simulink model "TV_2017"  (R2016a)
settings: Solver=FixedStepAuto  StartTime=0.0  StopTime=inf  FixedStep=0.001  RelTol=1e-3
PreLoadFcn:
  | TV_2017_parameters
values from neighbouring files (symbols this model uses):
  battery_voltage = single(530)    [HIL_parameters.m]    (also in HIL_parameters_2018.m; TV_2017_parameters.m; TV_2017_parameters_VD.m)
  car_params = Simulink_Car_params    [HIL_parameters.m]    (also in HIL_parameters_2018.m; TV_2017_parameters.m; TV_2017_parameters_VD.m)
  i_Diff = 16    [HIL_parameters.m]    (also in HIL_parameters_2018.m; TV_2017_parameters.m)
  Kp = 1    [HIL_parameters.m]    (also in HIL_parameters_2018.m; TV_2017_parameters.m; TV_2017_parameters_VD.m)
  motor_data = struct    [HIL_parameters.m]    (also in HIL_parameters_2018.m; TV_2017_parameters.m)
  powerLimitControl = Simulink_el    [HIL_parameters.m]    (also in HIL_parameters_2018.m; TV_2017_parameters.m; TV_2017_parameters_VD.m)
  settings = Simulink_Settings    [HIL_parameters.m]    (also in HIL_parameters_2018.m; TV_2017_parameters.m; TV_2017_parameters_VD.m)
  SpdC_BCC = 0    [HIL_parameters.m]    (also in HIL_parameters_2018.m; TV_2017_parameters.m; TV_2017_parameters_VD.m)
  Speed_Neg_sat = -21    [HIL_parameters.m]    (also in HIL_parameters_2018.m; TV_2017_parameters.m; TV_2017_parameters_VD.m)
  Speed_Pos_sat = 21    [HIL_parameters.m]    (also in HIL_parameters_2018.m; TV_2017_parameters.m; TV_2017_parameters_VD.m)
  SteeringAngleFL = [-23.80 -22.65 -21.50 -20.34 -19.18 -18.03 -16.86 -15.70 -14.53 -13.35 -12.18 -10.99 -9.80 -8.61 -7.40 -6.19 -4.97 -3.75 -2.51 -1.26 0 1.27 2.56 3.85 5.17 6.50 7.84 9.21 10.59 12.00 13.42 14.88 16.36 17.87 19.41 20.99 22.61 24.26 25.97 27.73 29.54]    [CarSetupAnalysis2018.m]    (also in HIL_parameters_2018.m; TV_2017_parameters.m; TV_2017_parameters_VD.m = [-24.129 -22.950 -21.772 -20.593 -19.413 -18.232 -17.050 -15)
  SteeringAngleFR = [-29.54 -27.73 -25.97 -24.26 -22.61 -20.99 -19.41 -17.87 -16.36 -14.88 -13.42 -12.00 -10.59 -9.21 -7.84 -6.50 -5.17 -3.85 -2.56 -1.27 0 1.26 2.51 3.75 4.97 6.19 7.40 8.61 9.80 10.99 12.18 13.35 14.53 15.70 16.86 18.03 19.18 20.34 21.50 22.65 23.80]    [CarSetupAnalysis2018.m]    (also in HIL_parameters_2018.m; TV_2017_parameters.m; TV_2017_parameters_VD.m = [-29.3050 -27.5340 -25.8140 -24.1410 -22.5110 -20.9180 -19.3)
  SteeringWhAngle = [-105 -99.75 -94.5 -89.25 -84 -78.75 -73.5 -68.25 -63 -57.75 -52.5 -47.25 -42 -36.75 -31.5 -26.25 -21.0 -15.75 -10.5 -5.25 0.0 5.25 10.50 15.75 21.00 26.25 31.50 36.75 42.00 47.25 52.50 57.75  63.00 68.25 73.50 78.75 84.00 89.25 94.50 99.75 105.00]    [TV_2017_parameters_VD.m]
  Tn_n = 0    [HIL_parameters.m]    (also in HIL_parameters_2018.m; TV_2017_parameters.m; TV_2017_parameters_VD.m)
  tractionControl = Simulink_tc    [HIL_parameters.m]    (also in HIL_parameters_2018.m; IterativeTractionControlTuning.m; TV_2017_parameters.m; TV_2017_parameters_VD.m)
  yawMomentGenerator = struct    [HIL_parameters.m]    (also in HIL_parameters_2018.m = Simulink_yawRate2; TV_2017_parameters.m = Simulink_yawRate2)
  yawRateControl = Simulink_yawRate    [HIL_parameters.m]    (also in HIL_parameters_2018.m; TV_2017_parameters.m; TV_2017_parameters_VD.m)
undefined symbols (not defined in the file or in its folder): DiscIntNeverNeededParam, magnitude, speedEstimation, TC_Decr_Gas, TC_Derivative, TC_Incr_Gas, TC_On, TC_Relay_Off, TC_Relay_On
libraries: CarMaker4SL x350, simulink_extras x63, simulink x37, dspfdesign x2
(part 8 of 14)

== system TV_2017/CarMaker/IPG Vehicle3/PowerTrain/Electric Powertrain/E-Gas // E-Motor/Electronic Gas Pedal RR/Subsystem1 ==
  VC.Gas : Inport
  E_Gas. : Inport  Port=2
  Car.LongSlip : Inport  Port=3
  Add : Sum
  Compare To Constant : simulink/Logic and Bit Operations/Compare To Constant  relop=>  const=TC_Derivative  OutDataTypeStr=uint8  ZeroCross=off
  Derivative : Derivative
  Fcn : Fcn  Expr=u >0.05
  Fcn1 : Fcn  Expr=u+TC_Incr_Gas
  Fcn2 : Fcn  Expr=u-TC_Decr_Gas
  Multiport Switch : MultiPortSwitch  DataPortOrder=Zero-based contiguous  zeroidx=on
  Relational Operator : RelationalOperator  Operator=<=  InputSameDT=on
  Relay : Relay  OnSwitchValue=TC_Relay_On  OffSwitchValue=TC_Relay_Off
  S-R Flip-Flop : simulink_extras/Flip Flops/S-R Flip-Flop  initial_condition=0
  Saturation : Saturate  UpperLimit=1  LowerLimit=0
  Saturation1 : Saturate  UpperLimit=1  LowerLimit=0
  Switch : Switch  Criteria=u2 > Threshold
  Terminator : Terminator
  E_Gas : Outport
  wires:
  Car.LongSlip/1 -> Relay/1, Derivative/1, Fcn/1
  Relay/1 -> Add/1
  Derivative/1 -> Compare To Constant/1
  Compare To Constant/1 -> Add/2
  Add/1 -> Multiport Switch/1
  Multiport Switch/1 -> E_Gas/1
  VC.Gas/1 -> Relational Operator/1, [A]
  E_Gas./1 -> Relational Operator/2, Fcn1/1, Fcn2/1, Multiport Switch/3
  S-R Flip-Flop/2 -> Terminator/1
  S-R Flip-Flop/1 -> Switch/2
  Switch/1 -> Multiport Switch/2
  Fcn/1 -> S-R Flip-Flop/1
  Relational Operator/1 -> S-R Flip-Flop/2
  Fcn1/1 -> Saturation1/1
  Saturation1/1 -> Switch/1
  Fcn2/1 -> Saturation/1
  Saturation/1 -> Multiport Switch/4
  [A] -> Switch/3

== matlab function TV_2017/CarMaker/Control_System /Yaw_rate_Mz_generator/Yaw Rate Controller /yawRateReference ==
  data: r_der_error output; r_error output; vx output; states input Bus: States; prev_r_error input; r_ref output; yawRateControl parameter; car_params parameter; r_lim output; settings parameter
function [r_der_error,r_error, vx, r_ref,r_lim]...
          = yawrate_reference(states,prev_r_error, yawRateControl, car_params,settings)

%#codegen
updatefactor = single(1);
r_lim = single(0);
delta = states.wheel_angle;
delta_der = states.wheel_speed;
% If Ku is negative there will be a problem if the denominator approaches
% zero at high speeds
r_ref = (states.V_x/(yawRateControl.r_ref_tuning_param + yawRateControl.Ku*states.V_x^2))*tan(delta); %  tan

%r_ref = (states.V_x/(yawRateControl.r_ref_tuning_param*(1 + yawRateControl.Ku*states.V_x^2)))* delta;

%Fzi = [states.Fz_FL states.Fz_FR states.Fz_RL states.Fz_RR];
if yawRateControl.enable_r_ref_limit == 1
    r_lim = settings.mu*yawRateControl.mu_scaling_r_ref_limit*9.81/states.V_x;
    if abs(r_ref) > abs(r_lim)
        r_ref = r_lim*sign(r_ref);
    end
end

r = states.r;
r_error = prev_r_error*(1-updatefactor) + updatefactor*(r_ref-r);
r_ref_der = (states.ax*delta + states.V_x*delta_der)/yawRateControl.r_ref_tuning_param;
r_der_error = r_ref_der*yawRateControl.ref_weight - states.r_der*yawRateControl.meas_weight;

vx = states.V_x;
end

== matlab function TV_2017/CarMaker/Control_System /Slip Rate Control /Traction Controllers/MATLAB Function1 ==
  data: states input Bus: States; SR_FL output; SR_FR output; SR_RL output; SR_RR output; T_req input; tractionControl parameter; Kp output; Ki output; settings parameter; T_tv input Bus: Ti_lim
function [SR_FL, SR_FR, SR_RL, SR_RR, Kp, Ki] = slipRatioAndGains(states, T_req, tractionControl, settings, T_tv)
%#codegen


SR_FL = states.SR_FL;
SR_FR = states.SR_FR;
SR_RL = states.SR_RL;
SR_RR = states.SR_RR;



if (states.V_x >= 0) 
    vx_kmh = states.V_x*3.6;
else
    vx_kmh = single(0);
end

    

a_kp = single((tractionControl.Kp_end - tractionControl.Kp_start) / tractionControl.lookup_speed_end_kmh);
a_ki = single((tractionControl.Ki_end - tractionControl.Ki_start) / tractionControl.lookup_speed_end_kmh);



if ( ( (T_req + 0.0001) > 0) && (vx_kmh < tractionControl.full_gain_limit_kmh) )   
    Kp = min( (a_kp*max(0,vx_kmh) + tractionControl.Kp_start), tractionControl.Kp_end)  * abs(T_req)/(settings.max_motor_torque*4);
    Ki = min( (a_ki*max(0,vx_kmh) + tractionControl.Ki_start), tractionControl.Ki_end)  * abs(T_req)/(settings.max_motor_torque*4);
else
    Kp = min( (a_kp*max(0,vx_kmh) + tractionControl.Kp_start), tractionControl.Kp_end);
    Ki = min( (a_ki*max(0,vx_kmh) + tractionControl.Ki_start), tractionControl.Ki_end);
end

end






% This one solves starting from 0 kmh with the driver controlling the
% throttle. This statement reduces the gains according to the requested
% torque, to avoid oscillating torque output


% if ( ( (T_req + 0.0001) > 0) && (vx_kmh < tractionControl.full_gain_limit_kmh) )   
%     Kp_driving = min( (a_kp*max(0,vx_kmh) + tractionControl.Kp_start), tractionControl.Kp_end)  * abs(T_req)/(settings.max_motor_torque*4);
%     Ki_driving = min( (a_ki*max(0,vx_kmh) + tractionControl.Ki_start), tractionControl.Ki_end)  * abs(T_req)/(settings.max_motor_torque*4);
%     Kp_FL = Kp_driving;
%     Kp_FR = Kp_driving;
%     Kp_RL = Kp_driving;
%     Kp_RR = Kp_driving;
%     
%     Ki_FL = Ki_driving;
%     Ki_FR = Ki_driving;
%     Ki_RL = Ki_driving;
%     Ki_RR = Ki_driving;
%     %Kp = min( (a_kp*max(0,vx_kmh) + tractionControl.Kp_start), tractionControl.Kp_end)  * abs(T_req)/(settings.max_motor_torque*4);
%     %Ki = min( (a_ki*max(0,vx_kmh) + tractionControl.Ki_start), tractionControl.Ki_end)  * abs(T_req)/(settings.max_motor_torque*4);
% 
% % T_req positive and speed over full gain limit
% elseif ( ( (T_req + 0.0001) > 0) && (vx_kmh > tractionControl.full_gain_limit_kmh))
%     Kp_driving = min( (a_kp*max(0,vx_kmh) + tractionControl.Kp_start), tractionControl.Kp_end);
%     Ki_driving = min( (a_ki*max(0,vx_kmh) + tractionControl.Ki_start), tractionControl.Ki_end);
%     Kp_FL = Kp_driving;
%     Kp_FR = Kp_driving;
%     Kp_RL = Kp_driving;
%     Kp_RR = Kp_driving;
%     
%     Ki_FL = Ki_driving;
%     Ki_FR = Ki_driving;
%     Ki_RL = Ki_driving;
%     Ki_RR = Ki_driving;    
% else   
%     Kp_FL = min( (a_kp*max(0,vx_kmh) + tractionControl.Kp_start), tractionControl.Kp_end);
%     Kp_FR = min( (a_kp*max(0,vx_kmh) + tractionControl.Kp_start), tractionControl.Kp_end);
%     Kp_RL = min( (a_kp*max(0,vx_kmh) + tractionControl.Kp_start), tractionControl.Kp_end);
%     Kp_RR = min( (a_kp*max(0,vx_kmh) + tractionControl.Kp_start), tractionControl.Kp_end);
%     
%     Ki_FL = min( (a_ki*max(0,vx_kmh) + tractionControl.Ki_start), tractionControl.Ki_end);
%     Ki_FR = min( (a_ki*max(0,vx_kmh) + tractionControl.Ki_start), tractionControl.Ki_end);
%     Ki_RL = min( (a_ki*max(0,vx_kmh) + tractionControl.Ki_start), tractionControl.Ki_end);
%     Ki_RR = min( (a_ki*max(0,vx_kmh) + tractionControl.Ki_start), tractionControl.Ki_end);
%     
%     %Kp = tractionControl.Kp_braking;
%     %Ki = tractionControl.Ki_braking;
% end
% 
% if ( (T_tv.FL < 0) || (T_tv.FR < 0) || (T_tv.RL < 0) || (T_tv.RR < 0) )
%     Kp = tractionControl.Kp_braking;
%     Ki = tractionControl.Ki_braking;
% end

== matlab function TV_2017/CarMaker/Control_System /MATLAB Function3 ==
  data: Ti input Bus: Ti_lim; states input; Ti_pos output Bus: Ti_pos; Ti_neg output Bus: Ti_neg; wi_setpoints output Bus: wi_set; settings parameter; car_params parameter; overTorque output
function [Ti_pos, Ti_neg, wi_setpoints, overTorque] = setPointCalculation(Ti,states,settings,car_params)
%#codegen

%Conversion factor to calculate RPM limits based on speed limits
%v_to_motor_RPM = single(60*car_params.GR/(2*pi*car_params.r_eff));
overTorque = int8(0);
r = car_params.r_eff;
GR = car_params.GR;
scale_factor = 5;
not_in_use = settings.RPM_scaling;
max_rpm = settings.max_RPM;
KERS_RPM_setpoint = settings.KERS_motor_RPM_setpoint;
%scaled_RPM_lim_pos = states.V_x* (60/2*pi*r)*scale_factor;
v_x = states.V_x;
if v_x>5;
    scaled_RPM_lim_pos =  min([max_rpm ,GR*v_x* (60/2*pi*r)*scale_factor]);
else
   scaled_RPM_lim_pos = single( min([max_rpm ,GR*5* (60/2*pi*r)*scale_factor]));
end


if max([Ti.FL Ti.FR Ti.RL Ti.RR]) > (21+0.0001)
    %this is bad
    overTorque = int8(1);
end



 %***************** FL *********** 

if  (Ti.FL <= 0)  
    Ti_pos.FL = int16(0);
    Ti_neg.FL = int16(max(-settings.max_motor_brake_torque/car_params.Mn, Ti.FL/car_params.Mn));
    wi_setpoints.FL = int16(KERS_RPM_setpoint);

elseif Ti.FL > 0
    Ti_pos.FL = int16(min(21/car_params.Mn , Ti.FL/car_params.Mn));
    Ti_neg.FL = int16(0);
    wi_setpoints.FL = int16(max_rpm);  
else
    Ti_pos.FL = int16(0);
    Ti_neg.FL = int16(0);
    wi_setpoints.FL = int16(1); 
end

%***************** FR ************

if  (Ti.FR <= 0)
    Ti_pos.FR = int16(0);
    Ti_neg.FR = int16(max(-settings.max_motor_brake_torque/car_params.Mn, Ti.FR/car_params.Mn));
    wi_setpoints.FR = int16(KERS_RPM_setpoint);

elseif Ti.FR > 0        
    Ti_pos.FR = int16( min(21/car_params.Mn , Ti.FR/car_params.Mn));
    Ti_neg.FR = int16(0);
    wi_setpoints.FR = int16(max_rpm);  
else
    Ti_pos.FR = int16(0);
    Ti_neg.FR = int16(0);
    wi_setpoints.FR = int16(1); 
end
%***************** RL ************
if  (Ti.RL <= 0)
    Ti_pos.RL = int16(0);
    Ti_neg.RL = int16(max(-settings.max_motor_brake_torque/car_params.Mn, Ti.RL/car_params.Mn));
    wi_setpoints.RL = int16(KERS_RPM_setpoint);

elseif Ti.RL > 0
    Ti_pos.RL = int16(min(21/car_params.Mn , Ti.RL/car_params.Mn));
    Ti_neg.RL = int16(0);
    wi_setpoints.RL = int16(max_rpm);  
else
    Ti_pos.RL = int16(0);
    Ti_neg.RL = int16(0);
    wi_setpoints.RL = int16(1); 
end

%***************** RR ************
if (Ti.RR <= 0)
    Ti_pos.RR = int16(0);
    Ti_neg.RR = int16(max(-settings.max_motor_brake_torque/car_params.Mn, Ti.RR/car_params.Mn));
    wi_setpoints.RR = int16(KERS_RPM_setpoint);

elseif Ti.RR > 0
    Ti_pos.RR = int16(min(21/car_params.Mn , Ti.RR/car_params.Mn));
    Ti_neg.RR = int16(0);
    wi_setpoints.RR = int16(max_rpm);  
else
    Ti_pos.RR = int16(0);
    Ti_neg.RR = int16(0);
    wi_setpoints.RR = int16(1); 
end
end



% _________________________________________________________________________________________  
% 
% %***************** FL ************
% if dynamic_rpm ==1
%     if  (Ti.FL <= 0)  
%         Ti_pos.FL = int16(0);
%         Ti_neg.FL = int16(max(-settings.max_motor_brake_torque/car_params.Mn, Ti.FL/car_params.Mn));
%         wi_setpoints.FL = int16(KERS_RPM_setpoint);
% 
%     elseif Ti.FL > 0 
%         Ti_pos.FL = int16( Ti.FL/car_params.Mn);
%         Ti_neg.FL = int16(0);
%         wi_setpoints.FL = int16(scaled_RPM_lim_pos);  
%     else
%         Ti_pos.FL = int16(0);
%         Ti_neg.FL = int16(0);
%         wi_setpoints.FL = int16(2); 
%     end
% 
%     %***************** FR ************
% 
%     if  (Ti.FR <= 0)
%         Ti_pos.FR = int16(0);
%         Ti_neg.FR = int16(max(-settings.max_motor_brake_torque/car_params.Mn, Ti.FR/car_params.Mn));
%         wi_setpoints.FR = int16(KERS_RPM_setpoint);
% 
%     elseif Ti.FR > 0
%         Ti_pos.FR = int16( Ti.FR/car_params.Mn);
%         Ti_neg.FR = int16(0);
%         wi_setpoints.FR = int16(scaled_RPM_lim_pos);  
%     else
%         Ti_pos.FR = int16(0);
%         Ti_neg.FR = int16(0);
%         wi_setpoints.FR = int16(2); 
%     end
%     %***************** RL ************
%     if  (Ti.RL <= 0)
%         Ti_pos.RL = int16(0);
%         Ti_neg.RL = int16(max(-settings.max_motor_brake_torque/car_params.Mn, Ti.RL/car_params.Mn));
%         wi_setpoints.RL = int16(KERS_RPM_setpoint);
% 
%     elseif Ti.RL > 0
%         Ti_pos.RL = int16( Ti.RL/car_params.Mn);
%         Ti_neg.RL = int16(0);
%         wi_setpoints.RL = int16(scaled_RPM_lim_pos);  
%     else
%         Ti_pos.RL = int16(0);
%         Ti_neg.RL = int16(0);
%         wi_setpoints.RL = int16(2); 
%     end
% 
%     %***************** RR ************
%     if (Ti.RR <= 0)
%         Ti_pos.RR = int16(0);
%         Ti_neg.RR = int16(max(-settings.max_motor_brake_torque/car_params.Mn, Ti.RR/car_params.Mn));
%         wi_setpoints.RR = int16(KERS_RPM_setpoint);
% 
%     elseif Ti.RR > 0
%         Ti_pos.RR = int16( Ti.RR/car_params.Mn);
%         Ti_neg.RR = int16(0);
%         wi_setpoints.RR = int16(scaled_RPM_lim_pos);  
%     else
%         Ti_pos.RR = int16(0);
%         Ti_neg.RR = int16(0);
%         wi_setpoints.RR = int16(2); 
%     end
%     
%     
% else
%     
%     
    
  % _________________________________________________________________________________________  
% % The RPM at which KERS is turned off
% RPM_limit_low = settings.KERS_speed_limit_hyst_low*v_to_motor_RPM;
% 
% % The RPM at which KERS is allowed again
% RPM_limit_high = settings.KERS_speed_limit_hyst_high*v_to_motor_RPM;
% 
% 
%    persistent firstIteration;
%    persistent KERS_ALLOWED_FL;
%    persistent KERS_ALLOWED_FR;
%    persistent KERS_ALLOWED_RL;
%    persistent KERS_ALLOWED_RR;
%    
%    
%    % Hysteresis on regenerative input based on RPM to avoid oscillation around 
%    % allowed KERS RPM 
%    if isempty(firstIteration)
%       firstIteration = 2; % Avoid overflow in the register and count 1 again
%       KERS_ALLOWED_FL = uint32(0);
%       KERS_ALLOWED_FR = uint32(0);
%       KERS_ALLOWED_RL = uint32(0);
%       KERS_ALLOWED_RR = uint32(0);
%    else
%        
%        %Hysteris around the minimum RPM Set point
%        if     ( (KERS_ALLOWED_FL == 0) && (states.RPM_FL > RPM_limit_high) )
%            KERS_ALLOWED_FL = uint32(1);
%        elseif ( (KERS_ALLOWED_FL == 1) && (states.RPM_FL < RPM_limit_low) )
%            KERS_ALLOWED_FL = uint32(0);
%        end
%        if     ( (KERS_ALLOWED_FR == 0) && (states.RPM_FR > RPM_limit_high) )
%            KERS_ALLOWED_FR = uint32(1);
%        elseif ( (KERS_ALLOWED_FR == 1) && (states.RPM_FR < RPM_limit_low) )
%            KERS_ALLOWED_FR = uint32(0);
%        end
%        if     ( (KERS_ALLOWED_RL == 0) && (states.RPM_RL > RPM_limit_high) )
%            KERS_ALLOWED_RL = uint32(1);
%        elseif ( (KERS_ALLOWED_RL == 1) && (states.RPM_RL < RPM_limit_low) )
%            KERS_ALLOWED_RL = uint32(0);
%        end
%        if     ( (KERS_ALLOWED_RR == 0) && (states.RPM_RR > RPM_limit_high) )
%            KERS_ALLOWED_RR = uint32(1);
%        elseif ( (KERS_ALLOWED_RR == 1) && (states.RPM_RR < RPM_limit_low) )
%            KERS_ALLOWED_RR = uint32(0);
%        end
%        
%        % Hysteresis around maximum RPM ? 
%        
%    end   
%       
% %***************** FL ************
% 
% if ( (Ti.FL <= 0) && (KERS_ALLOWED_FL == 1) ) 
%     Ti_pos.FL = int16(0);
%     Ti_neg.FL = int16( Ti.FL/car_params.Mn);
%     wi_setpoints.FL = int16(KERS_RPM_setpoint);
% elseif ( (Ti.FL <= 0) && (KERS_ALLOWED_FL == 0) )
%     Ti_pos.FL = int16(0);
%     Ti_neg.FL = int16(0);
%     wi_setpoints.FL = int16(0);
% elseif Ti.FL > 0
%     Ti_pos.FL = int16( Ti.FL/car_params.Mn);
%     Ti_neg.FL = int16(0);
%     wi_setpoints.FL = int16(max_rpm);  
% else
%     Ti_pos.FL = int16(0);
%     Ti_neg.FL = int16(0);
%     wi_setpoints.FL = int16(0); 
% end
% 
% %***************** FR ************
% 
% if ( (Ti.FR <= 0) && (KERS_ALLOWED_FR == 1) ) 
%     Ti_pos.FR = int16(0);
%     Ti_neg.FR = int16( Ti.FR/car_params.Mn);
%     wi_setpoints.FR = int16(KERS_RPM_setpoint);
% elseif ( (Ti.FR <= 0) && (KERS_ALLOWED_FR == 0) )
%     Ti_pos.FR = int16(0);
%     Ti_neg.FR = int16(0);
%     wi_setpoints.FR = int16(0);
% elseif Ti.FR > 0
%     Ti_pos.FR = int16( Ti.FR/car_params.Mn);
%     Ti_neg.FR = int16(0);
%     wi_setpoints.FR = int16(max_rpm);  
% else
%     Ti_pos.FR = int16(0);
%     Ti_neg.FR = int16(0);
%     wi_setpoints.FR = int16(0); 
% end
% %***************** RL ************
% if ( (Ti.RL <= 0) && (KERS_ALLOWED_RL == 1) ) 
%     Ti_pos.RL = int16(0);
%     Ti_neg.RL = int16( Ti.RL/car_params.Mn);
%     wi_setpoints.RL = int16(KERS_RPM_setpoint);
% elseif ( (Ti.RL <= 0) && (KERS_ALLOWED_RL == 0) )
%     Ti_pos.RL = int16(0);
%     Ti_neg.RL = int16(0);
%     wi_setpoints.RL = int16(0);
% elseif Ti.RL > 0
%     Ti_pos.RL = int16( Ti.RL/car_params.Mn);
%     Ti_neg.RL = int16(0);
%     wi_setpoints.RL = int16(max_rpm);  
% else
%     Ti_pos.RL = int16(0);
%     Ti_neg.RL = int16(0);
%     wi_setpoints.RL = int16(0); 
% end
% 
% %***************** RR ************
% if ( (Ti.RR <= 0) && (KERS_ALLOWED_RR == 1) ) 
%     Ti_pos.RR = int16(0);
%     Ti_neg.RR = int16( Ti.RR/car_params.Mn);
%     wi_setpoints.RR = int16(KERS_RPM_setpoint);
% elseif ( (Ti.RR <= 0) && (KERS_ALLOWED_RR == 0) )
%     Ti_pos.RR = int16(0);
%     Ti_neg.RR = int16(0);
%     wi_setpoints.RR = int16(0);
% elseif Ti.RR > 0
%     Ti_pos.RR = int16( Ti.RR/car_params.Mn);
%     Ti_neg.RR = int16(0);
%     wi_setpoints.RR = int16(max_rpm);  
% else
%     Ti_pos.RR = int16(0);
%     Ti_neg.RR = int16(0);
%     wi_setpoints.RR = int16(0); 
% end
% 
% end

== matlab function TV_2017/CarMaker/Control_System /Yaw_rate_Mz_generator/Yaw Rate Controller /gainScheduling ==
  data: Kd output; vx_kmh input; Kp output; Ki output; yawRateControl parameter
function [Kd, Kp, Ki] = gainScheduling(vx_kmh,yawRateControl)
%#codegen
if (vx_kmh <= 0)
    vx_kmh = single(0);
end


% a_kp = single((yawRateControl.Kp_end - yawRateControl.Kp_start) / yawRateControl.lookup_speed_end_kmh);
% a_ki = single((yawRateControl.Ki_end - yawRateControl.Ki_start) / yawRateControl.lookup_speed_end_kmh);
% a_kd = single((yawRateControl.Kd_end - yawRateControl.Kd_start) / yawRateControl.lookup_speed_end_kmh);
% 
% if (vx_kmh <= 0)
%     vx_kmh = single(0);
% end
% 
% Kp = min( (a_kp*max(0.1,vx_kmh) + yawRateControl.Kp_start), yawRateControl.Kp_end);
% 
% Ki = min( (a_ki*max(0.1,vx_kmh) + yawRateControl.Ki_start), yawRateControl.Ki_end);
% 
% Kd = min( (a_kd*max(0.1,vx_kmh) + yawRateControl.Kd_start), yawRateControl.Kd_end);
% 
% end

Kp_values = [yawRateControl.Kp_start yawRateControl.Kp_start  yawRateControl.Kp_end yawRateControl.Kp_end];
Kp_speeds = [0 yawRateControl.lookup_speed_end_kmh (yawRateControl.lookup_speed_end_kmh+20)  115];

Ki_values = [yawRateControl.Ki_start yawRateControl.Ki_start  yawRateControl.Ki_end yawRateControl.Ki_end];
Ki_speeds = [0 yawRateControl.lookup_speed_end_kmh (yawRateControl.lookup_speed_end_kmh+20)  115];

Kd_values = [yawRateControl.Kd_start yawRateControl.Kd_start  yawRateControl.Kd_end yawRateControl.Kd_end];
Kd_speeds = [0 yawRateControl.lookup_speed_end_kmh (yawRateControl.lookup_speed_end_kmh+20)  115];


Kp = interp1(Kp_speeds,Kp_values,vx_kmh); 
Ki = interp1(Ki_speeds,Ki_values,vx_kmh);
Kd = interp1(Kd_speeds,Kd_values,vx_kmh);


if Kp>= 0
    Kp = Kp;
elseif Kp < 0 
    Kp = Kp;
else
    Kp = single(0);
end

if Ki>= 0
    Ki = Ki;
elseif Ki < 0 
    Ki = Ki;
else
    Ki = single(0);
end

if Kd>= 0
    Kd = Kd;
elseif Kd < 0 
    Kd = Kd;
else
    Kd = single(0);
end



breakpoint = 1;

== matlab function TV_2017/CarMaker/Control_System /Subsystem/OutputTelemetri ==
  data: states input; OutputTelemetri_control output Bus: OutputTelemetri_Control; T_req input; r_ref input; Mz_ref_to_telemetry input
function OutputTelemetri_control = OutputTelemetri(states, T_req, r_ref, Mz_ref_to_telemetry)
%#codegen

OutputTelemetri_control.T_req   = T_req;
OutputTelemetri_control.Mz_ref  = Mz_ref_to_telemetry;
OutputTelemetri_control.r_ref   = r_ref;
end

== matlab function TV_2017/CarMaker/Control_System /Subsystem/Torque allocation 2017/Inverter temperature limiter ==
  data: states input; maxMotorTorque output Bus: maxMotorTorque; settings parameter; car_params parameter
function maxMotorTorque = maxMotorTorque_InvTemp(states,settings, car_params)
%#codegen
inv_FL_temp =int16(20);
inv_FR_temp =20;
inv_RL_temp =20;
inv_RR_temp =20;


% The inverters limits output torque based on internal temperature
mmt                 =  single(settings.max_motor_torque);
upper_max_temp      =  single(car_params.AMK_inverter_upper_max_temp);
cutoff_temp         =  single(car_params.AMK_inverter_cutoff_temp);

torque = [mmt, mmt, single(0)]; %breakpoints for lookup function
temp = [single(0), upper_max_temp, cutoff_temp];

inv_FL_temp = single(states.AMK_inverter_temp_FL);
inv_FR_temp = single(states.AMK_inverter_temp_FR);
inv_RL_temp = single(states.AMK_inverter_temp_RL);
inv_RR_temp = single(states.AMK_inverter_temp_RR);

%  y = interp1(xdata,ydata,x)
maxMotorTorque.mmt_FL = interp1(  temp , torque,  inv_FL_temp  );
maxMotorTorque.mmt_FR = interp1(  temp , torque,  inv_FR_temp  );
maxMotorTorque.mmt_RL = interp1(  temp , torque,  inv_RL_temp  );
maxMotorTorque.mmt_RR = interp1(  temp , torque,  inv_RR_temp  );

== matlab function TV_2017/CarMaker/ECU input Sensors /estimated "Measured Power" based on Torque, RPM and datasheet IRL this is measured/MATLAB Function ==
  data: RPM_FL_IN input; RPM_FR_IN input; RPM_RL_IN input; RPM_RR_IN input; Pm_FL output; T input; T_FL output; RPM_FL output; Pm_FR output; T_FR output; RPM_FR output; Pm_RL output; T_RL output; RPM_RL output; Pm_RR output; T_RR output; RPM_RR output
function [Pm_FL, T_FL, RPM_FL,Pm_FR, T_FR, RPM_FR,Pm_RL, T_RL,...
          RPM_RL,Pm_RR, T_RR, RPM_RR] = powerMeasurement(RPM_FL_IN, RPM_FR_IN,RPM_RL_IN,RPM_RR_IN, T)
%#codegen

%Conversion from RPM to rad/s
c = single(2*pi/60);

T_FL = T.FL;
T_FR = T.FR;
T_RL = T.RL;
T_RR = T.RR;

RPM_FL = RPM_FL_IN;
RPM_FR = RPM_FR_IN;
RPM_RL = RPM_RL_IN;
RPM_RR = RPM_RR_IN;


Pm_FL = RPM_FL*c*T.FL;
Pm_FR = RPM_FR*c*T.FR;
Pm_RL = RPM_RL*c*T.RL;
Pm_RR = RPM_RR*c*T.RR;

== matlab function TV_2017/CarMaker/Control_System /Subsystem/Torque allocation 2016/MATLAB Function ==
  data: states input; maxMotorTorque output Bus: maxMotorTorque; settings parameter
function maxMotorTorque = findMaxMotorTorque(states,settings)
%#codegen

% DC Voltage                             / states
% Max allowable current draw in total    /settings
% Load distribution                      /states

Fzi = [max(1,states.Fz_FL) max(1,states.Fz_FR) max(1,states.Fz_RL) max(1,states.Fz_RR)]';

switch settings.TV_Method
    case 1 % No negative torque
        alfa_r =  (Fzi(3) + Fzi(4)) / (Fzi(1) + Fzi(2) + Fzi(3) + Fzi(4));
    case 2 % with negative torque
        alfa_r =  (Fzi(3) + Fzi(4)) / (Fzi(1) + Fzi(2) + Fzi(3) + Fzi(4));
    case 3 % static 25 %
        alfa_r = single(0.5);
    case 4 % with negative torque, no Fz
        alfa_r = single(0.5);
    otherwise
        alfa_r = single(0.5);
end

RPM_to_angular = single(2*pi/60);
omega_FL = states.RPM_FL*RPM_to_angular;
omega_FR = states.RPM_FR*RPM_to_angular;
omega_RL = states.RPM_RL*RPM_to_angular;
omega_RR = states.RPM_RR*RPM_to_angular;

mmt = settings.max_motor_torque;
available_power = states.DC_voltage*settings.max_battery_discharge;

max_torque_front = min(mmt, (available_power*(1-alfa_r))/ (2 * max( max(1,omega_FL), max(1,omega_FR))) );
max_torque_rear = min(mmt, (available_power*alfa_r)     / (2 * max( max(1,omega_RL), max(1,omega_RR))) );
                      
maxMotorTorque.mmt_FL = max_torque_front;
maxMotorTorque.mmt_FR = max_torque_front;
maxMotorTorque.mmt_RL = max_torque_rear;
maxMotorTorque.mmt_RR = max_torque_rear;
maxMotorTorque.kers_allowed = single(0);

== matlab function TV_2017/CarMaker/Estimations/EstimateVx/velocity_Estimation ==
  data: sensors input Bus: SensorInputs; V_est_x output; normalForces input Bus: normalForces; settings parameter; car_params parameter; speedEstimation parameter
function V_est_x  = velocityEstimation(sensors,normalForces,settings,car_params,speedEstimation)
%#codegen


persistent firstIteration;
persistent v;
persistent error;
persistent K;
persistent drift;

k_FL = single(0); % Gain 
k_FR = single(0); % Gain
k_RL = single(0); % Gain
k_RR = single(0); % Gain
% Gains for trusting, not trusting wheel speed measurements
Hg = speedEstimation.High_gain;
Lg = speedEstimation.Low_gain;
% Variances
all_Var = single(0); % Variance for all measurements
front_rear_Var = single(0);
front_Var = single(0);
rear_Var = single(0);
left_Var = single(0);
right_Var = single(0);
% LIMITS:
velocity_deviation_limit = speedEstimation.velocity_deviation_limit;
lim = speedEstimation.variance_limit;
RPM_derivative_limit = speedEstimation.RPM_derivative_limit;

% Measurement vector
C = [1;1;1;1]; % Create four copies of predicted vx


c = single(2*pi/(car_params.GR*60));

t = settings.control_system_sample_time;
%Weights taken from wikipedia
%sg_Weight = single( [ 1; -8; 0; 8; -1] );
sg_Weight = single( [ -1; 8; 0; -8; 1] );
%sg_Weight = single([0.3; 0.1; -0.1 ; -0.3]);
%sg_Weight = single([1; -1; 0 ; -0]);
% ------------------------------
% COPY VARIABLES EACH TIMESTEP
% ------------------------------
S = sensors.steering_wheel_angle; % Steering angle in rad( Mean of front wheels)
ax = sensors.ax; % Should be true linear acceleration compensated for roll angle
%Fz, used to determine what wheel speeds to trust.
Fz = [normalForces.FL, normalForces.FR, normalForces.RL ,normalForces.RR];
% Determine CoG Vx from motor RPM. Simple atm. Not considering vy.
Whl_v_FL = sensors.RPM_FL*c*car_params.r_eff*cos(S) + sensors.yawRate*car_params.t_f;
Whl_v_FR = sensors.RPM_FR*c*car_params.r_eff*cos(S) - sensors.yawRate*car_params.t_f;
Whl_v_RL = sensors.RPM_RL*c*car_params.r_eff + sensors.yawRate*car_params.t_r;
Whl_v_RR = sensors.RPM_RR*c*car_params.r_eff - sensors.yawRate*car_params.t_r;
whl_speed.v_FL = Whl_v_FL;
whl_speed.v_FR = Whl_v_FR;
whl_speed.v_RL = Whl_v_RL;
whl_speed.v_RR = Whl_v_RR;


RPM = [sensors.RPM_FL, sensors.RPM_FR, sensors.RPM_RL, sensors.RPM_RR]';
% Measurement vector, compensated RPMS
Y_meas = [Whl_v_FL, Whl_v_FR, Whl_v_RL, Whl_v_RR]';
% Input Derivative of RPM
rateRPM_FL = sensors.RPM_der_FL;
rateRPM_FR = sensors.RPM_der_FR;
rateRPM_RL = sensors.RPM_der_RL;
rateRPM_RR = sensors.RPM_der_RR;

% Different sums of normal forces, used to determine what wheels to trust
left_Fz = sum(Fz([1 3]));
right_Fz = sum(Fz([2 4]));
front_Fz = sum(Fz(1:2));
rear_Fz = sum(Fz(3:4));
% ALGORITHM
if (isempty(firstIteration))
    K = single(ones(1,4));
    v = single(0);
    V_est_x = v;
    error = Y_meas- C*v;
    firstIteration = 2;
    drift = single(0);
else
    v_ins = sensors.V_x_INS + 0.05 + drift;
    mean_WhlV = max(0.001,mean(Y_meas));
    mean_front_WhlV = max(0.001,mean(Y_meas(1:2)));
    mean_rear_WhlV  = max(0.001,mean(Y_meas(3:4)));
    mean_left_WhlV  = max(0.001,mean(Y_meas([1 3])));
    mean_right_WhlV = max(0.001,mean(Y_meas([2 4])));

    all_Var = var(Y_meas,1)/mean_WhlV;
    front_rear_Var = var([mean_front_WhlV, mean_rear_WhlV],1)/mean_WhlV;
    front_Var = var(Y_meas(1:2),1)/mean_front_WhlV;
    rear_Var  = var(Y_meas(3:4),1)/mean_rear_WhlV;
    
    left_Var    = var(Y_meas([1 3]),1)/mean_left_WhlV;
    right_Var   = var(Y_meas([2 4]),1)/mean_right_WhlV;   
    
    if ( (abs(Whl_v_FL - v_ins) > velocity_deviation_limit)...
       && (abs(Whl_v_FR - v_ins) > velocity_deviation_limit)...
       && (abs(Whl_v_RL - v_ins) > velocity_deviation_limit)...
       && (abs(Whl_v_RR - v_ins) > velocity_deviation_limit) )
        
        K = [Lg, Lg, Lg, Lg];
    elseif (all_Var  < lim ) 
        % low variance for all wheels.
        % Check derivative of motor RPM
        if ( (rateRPM_FL > RPM_derivative_limit) ||...
             (rateRPM_FR > RPM_derivative_limit) ||...
             (rateRPM_RL > RPM_derivative_limit) ||...
             (rateRPM_RR > RPM_derivative_limit))
            K = [Lg, Lg, Lg, Lg];
        % Rate of change of RPM can be low but slip rate is large
        % Check against drifting INS velocity 
        else
            K = [Hg, Hg ,Hg ,Hg];
        end
    % Variance is high. What wheel(s) are causing this.. 
    % STRUCTURE:
    % 1 = FRONT AND REAR DIFFER
    % 2 = LEFT AND RIGHT DIFFER
    % 3 = FL WRONG
    % 4 = FR WRONG
    % 5 = RL WRONG
    % 6 = RR WRONG
    % 7 Combinations of 3-6 that are not handled in 1-2.
    
    %1: FRONT AND REAR DIFFER
    elseif( (right_Var > front_Var) && (right_Var > rear_Var)...
            && (left_Var > front_Var) && (left_Var > rear_Var))
        % High variance between front and rear, and low variance 
        % at front and rear.
        
        % Also need to check if front/rear wheels are slippin    
        % Front wheels over limit while rear is ok
        if (((rateRPM_FL > RPM_derivative_limit) ||...
             (rateRPM_FR > RPM_derivative_limit)) &&...
            ((rateRPM_RL < RPM_derivative_limit) ||...
             (rateRPM_RR < RPM_derivative_limit)) )
             
            K = [Lg, Lg, Hg, Hg];
        % Rear wheels over limit while front is ok
        elseif ( ((rateRPM_FL < RPM_derivative_limit) ||...
                 (rateRPM_FR < RPM_derivative_limit)) &&...
                ((rateRPM_RL > RPM_derivative_limit) ||...
                 (rateRPM_RR > RPM_derivative_limit)) )
             K = [Hg, Hg, Lg, Lg];
        % All are over limit
        elseif  ((rateRPM_FL > RPM_derivative_limit) &&...
                 (rateRPM_FR > RPM_derivative_limit) &&...
                 (rateRPM_RL > RPM_derivative_limit) &&...
                 (rateRPM_RR > RPM_derivative_limit) ) 
              K = [Lg, Lg, Lg, Lg];
              
        % The rate of change of RPM will flatten out and the high
        % slip ratio will still exist. Handle this
        
        % Check big difference in wheel speeds
        % Two cases. Driving and braking. 
        
        % Driving. Need logic to determine driving/braking
        elseif ( (RPM(1) + RPM(2)) > (RPM(3) + RPM(4)) )
            K = [Lg, Lg, Hg, Hg];
        elseif ( (RPM(1) + RPM(2)) < (RPM(3) + RPM(4)) )
            K = [Hg, Hg, Lg, Lg];
            % If frontFZ - rearFZ < 0, then FL is set to 0
            % Else it is set to a positive gain
%             k_FL = (1/abs(front_Fz-rear_Fz))*max(0,front_Fz - rear_Fz);
%             k_FR = (1/abs(front_Fz-rear_Fz))*max(0,front_Fz - rear_Fz);
% 
%             k_RL = (1/abs(rear_Fz-front_Fz))*max(0,rear_Fz-front_Fz)*0.5;
%             k_RR = (1/abs(rear_Fz-front_Fz))*max(0,rear_Fz-front_Fz)*0.5;
%            K = [k_FL, k_FR, k_RL, k_RR];
        end
    %2: LEFT AND RIGHT WHEELS DIFFER
    elseif ( ((front_Var > right_Var) && (rear_Var > right_Var)) ||...
            ( (front_Var > left_Var) && (rear_Var > left_Var)))
   
        k_FL = (1/abs(left_Fz-right_Fz))*max(0,left_Fz - right_Fz);
        k_RL = (1/abs(left_Fz-right_Fz))*max(0,left_Fz - right_Fz);
        
        k_FR = (1/abs(right_Fz-left_Fz))*max(0,right_Fz-left_Fz);
        k_RR = (1/abs(right_Fz-left_Fz))*max(0,right_Fz-left_Fz);
        
        K = [k_FL, k_FR, k_RL, k_RR];
        
    %3: FL WRONG
    elseif ( (left_Var > rear_Var) && (left_Var > right_Var)...
            && (front_Var > rear_Var) )
        k_FL = single(0);
        k_FR = single(0);
        k_RL = single(1);
        k_RR = single(1);
        K = [k_FL, k_FR, k_RL, k_RR];
    %4: FR WRONG
    elseif ( (right_Var > rear_Var) && (right_Var > left_Var)...
            && (front_Var > rear_Var))
        k_FL = single(0);
        k_FR = single(0);
        k_RL = single(1);
        k_RR = single(1);
        K = [k_FL, k_FR, k_RL, k_RR]; 
    %5: RL WRONG
    elseif ( (left_Var > front_Var) && (left_Var > right_Var)...
            && (rear_Var > front_Var))
        
        k_FL = single(1);
        k_FR = single(1);
        k_RL = single(0);
        k_RR = single(0);
        K = [k_FL, k_FR, k_RL, k_RR]; 
        
    %5: RR WRONG    
    elseif ( (right_Var > front_Var) && (right_Var > left_Var)...
            && (rear_Var > front_Var))
        k_FL = single(1);
        k_FR = single(1);
        k_RL = single(0);
        k_RR = single(0);
        K = [k_FL, k_FR, k_RL, k_RR]; 
    else
        k_FL = single(0);
        k_FR = single(0);
        k_RL = single(0);
        k_RR = single(0);
        K = [k_FL, k_FR, k_RL, k_RR]; 
    end
    
    drift = drift + 0.03*t;
   
    %v = v + t*ax;
    v = v + t*(ax + K*error);
    error = Y_meas - C*v ;
    V_est_x = 0.98*v;
end
end

== matlab function TV_2017/CarMaker/Control_System /Throttle // Brake Mapping ==
  data: states input; settings parameter; T_req output; car_params parameter
function T_req = pedalMapping(states,settings,car_params)
%#codegen

    KERS_pos = states.KERS_pos;
    throttle = min(1,states.Input_throttle);
    T_req = single(0);
    Fx_req = single(0);
    max_drive_torque = settings.max_motor_torque*4;
    max_brake_torque = settings.max_motor_brake_torque*4;
    
   persistent firstIteration;
   persistent KERS_allowed;
   
   % Hysteresis on KERS pedal input to avoid oscillation around 
   % allowed KERS speed. 
   if isempty(firstIteration)
      firstIteration = 2; %
      KERS_allowed = uint32(0);
   else
      % Hysteresis around the minimum KERS speed
       if     ( (KERS_allowed == 0) && (states.V_x > settings.KERS_speed_limit_hyst_high) )
           KERS_allowed = uint32(1);
       elseif ( (KERS_allowed == 1) && (states.V_x < settings.KERS_speed_limit_hyst_low) )
           KERS_allowed = uint32(0);
       end          
   end   
  if (settings.KERS_active == 1) 
      T_req = max_drive_torque*throttle  -  max_brake_torque*KERS_pos * single(KERS_allowed) ;
  else
      T_req = max_drive_torque*throttle ;
  end  
end

== matlab function TV_2017/CarMaker/Estimations/Fz_estimators/Fz_Estimation_acceleration based/Fz_acc_est ==
  data: sensors input Bus: SensorInputs; Fz_acc_est output Bus: normalForces; car_params parameter; alfa_r_acc output
function [Fz_acc_est, alfa_r_acc] =  FzEstAcc(sensors , car_params)
%#codegen
g = 9.81;
ax = sensors.ax;
ay = sensors.ay;

total_mass = 245;
sprung_mass = 124+70;
unsprung_front = car_params.unsprung_mass_per_wheel_newton_front;
unspring_rear = car_params.unsprung_mass_per_wheel_newton_rear;
cg_z = 0.300;%car_params.CoG_height;
t_f = car_params.t_f;
t_r = car_params.t_r;
l_f = car_params.l_f;%Distance CoG to front axle
l_r = car_params.l_r;%Distance CoG to rear axle

K_ax = 1.25;
K_ay = 1.20;

%estimate forces from spring, damper and ARB
Fz_acc_est.FL = g*sprung_mass*0.25 + unsprung_front - K_ax*0.25*ax*sprung_mass*cg_z/l_f - K_ay*0.25*ay*sprung_mass*cg_z/t_f;
Fz_acc_est.FR = g*sprung_mass*0.25 + unsprung_front - K_ax*0.25*ax*sprung_mass*cg_z/l_f + K_ay*0.25*ay*sprung_mass*cg_z/t_f;
Fz_acc_est.RL = g*sprung_mass*0.25 + unspring_rear  + K_ax*0.25*ax*sprung_mass*cg_z/l_r - K_ay*0.25*ay*sprung_mass*cg_z/t_r;
Fz_acc_est.RR = g*sprung_mass*0.25 + unspring_rear  + K_ax*0.25*ax*sprung_mass*cg_z/l_r + K_ay*0.25*ay*sprung_mass*cg_z/t_r;

alfa_r_acc = (1.5+ax/g)/(3);

== matlab function TV_2017/CarMaker/Estimations/Subsystem/SR_Calculation/Slip ratio ==
  data: V_x input; SR output Bus: SR; whl_v input Bus: Whl_speed; sensor input; car_params parameter
function SR = slipRatioCalculation(V_x,whl_v,sensor,car_params)
%#codegen

vx_to_wheel_factor = single(0.6);
vx_omega = sensor.yawRate*vx_to_wheel_factor;

Vx_FL = -vx_omega + V_x;
Vx_FR =  vx_omega + V_x;
Vx_RL = -vx_omega + V_x;
Vx_RR =  vx_omega + V_x;


SR.FL = single((whl_v.FL - Vx_FL) / max([1, abs(Vx_FL)]));    
SR.FR = single((whl_v.FR - Vx_FR) / max([1, abs(Vx_FR)]));
SR.RL = single((whl_v.RL - Vx_RL) / max([1, abs(Vx_RL)]));
SR.RR = single((whl_v.RR - Vx_RR) / max([1, abs(Vx_RR)]));

end

== matlab function TV_2017/CarMaker/Estimations/RPM_to_linearVelocity/whl_v_calculation ==
  data: sensors input Bus: SensorInputs; meanWheelAngle input; car_params parameter; whl_speed output Bus: Whl_speed
function whl_speed = rpmToWhlVelocity(sensors,meanWheelAngle,car_params)
%#codegen

S = meanWheelAngle; % Steering angle in rad( Mean of front wheels)
c = single(2*pi/(car_params.GR*60));

% Determine CoG Vx from motor RPM. Simple atm. Not considering vy.
whl_speed.FL = sensors.RPM_FL*c*car_params.r_eff*cos(S) ;%+ sensors.yawRate*car_params.t_f;
whl_speed.FR = sensors.RPM_FR*c*car_params.r_eff*cos(S) ;%- sensors.yawRate*car_params.t_f;
whl_speed.RL = sensors.RPM_RL*c*car_params.r_eff        ;%+ sensors.yawRate*car_params.t_r;
whl_speed.RR = sensors.RPM_RR*c*car_params.r_eff        ;%- sensors.yawRate*car_params.t_r;

== matlab function TV_2017/CarMaker/Estimations/Fx_Estimation/EstimateFx ==
  data: car_params parameter; Fx output Bus: Fx; sensors input Bus: SensorInputs; T_motor output Bus: T_motor
function [Fx, T_motor] = estimateFx(car_params, sensors)
%#codegen
Iq_FL = sensors.Iq_FL;
Iq_FR = sensors.Iq_FR;
Iq_RL = sensors.Iq_RL;
Iq_RR = sensors.Iq_RR;

Id_FL = sensors.Id_FL;
Id_FR = sensors.Id_FR;
Id_RL = sensors.Id_RL;
Id_RR = sensors.Id_RR;

Kt = car_params.Kt;     % Torque constant
Lq = car_params.Lq;     % Quadrature axis inductance 
Ld = car_params.Ld;     % Direct access inductance
Jw = car_params.Jw;     % Motor inertia
R  = car_params.r_eff;  % Radius center of rim to tire contact
GR = car_params.GR;     % Gear ratio
% Convert RPM Derivative to angular acceleration
c = single(2*pi/(GR*60));
ang_acc_FL = c*sensors.RPM_der_FL;
ang_acc_FR = c*sensors.RPM_der_FR;
ang_acc_RL = c*sensors.RPM_der_RL;
ang_acc_RR = c*sensors.RPM_der_RR;

% T_motor.FL = (Iq_FL*Kt*sqrt(2)-(Lq-Ld)*Id_FL);
% T_motor.FR = (Iq_FR*Kt*sqrt(2)-(Lq-Ld)*Id_FR);
% T_motor.RL = (Iq_RL*Kt*sqrt(2)-(Lq-Ld)*Id_RL);
% T_motor.RR = (Iq_RR*Kt*sqrt(2)-(Lq-Ld)*Id_RR);

T_motor.FL = (Iq_FL*Kt);
T_motor.FR = (Iq_FR*Kt);
T_motor.RL = (Iq_RL*Kt);
T_motor.RR = (Iq_RR*Kt);
%T_FL = T_CM.FL;
%T_FR = T_CM.FR;
%T_RL = T_CM.RL;
%T_RR = T_CM.RR;


Fx.FL = (T_motor.FL*GR - Jw*ang_acc_FL)/R;
Fx.FR = (T_motor.FR*GR - Jw*ang_acc_FR)/R;
Fx.RL = (T_motor.RL*GR - Jw*ang_acc_RL)/R;
Fx.RR = (T_motor.RR*GR - Jw*ang_acc_RR)/R;

== matlab function TV_2017/CarMaker/Estimations/friction_estimation/estimateFrictionCoefficient ==
  data: Fx input Bus: Fx; mu output; mu_estimate output; Fz input Bus: normalForces; SR input Bus: SR; settings parameter; normLongTireForce output Bus: normLongTireForce
function [mu, mu_estimate, normLongTireForce]= estimateFrictionCoefficient(Fx,Fz,SR,settings)
%#codegen
persistent mu_FL;
persistent mu_FR;
persistent mu_RL;
persistent mu_RR;
persistent firstIteration;

mu_forget_factor = 0.001;  %kan legges in som parameter etter hvert. (Emil.17.10.2017)
mu_growth_factor = 0.0001;
mu_shrink_factor = 0.0001;
mu_full_slip_lim = 0.23;
mu_hi_slip_lim   = 0.13;
mu_lo_slip_lim   = 0.09;
mu_no_slip_lim   = 0.05;


if isempty(firstIteration)
    firstIteration = 2; %
    mu_FL = settings.mu;
    mu_FR = settings.mu;
    mu_RL = settings.mu;
    mu_RR = settings.mu;
    normLongTireForce.FL = single(0);
    normLongTireForce.FR = single(0);
    normLongTireForce.RL = single(0);
    normLongTireForce.RR = single(0);
   
      
else
    normLongTireForce.FL = (Fx.FL/Fz.FL);
    normLongTireForce.FR = (Fx.FR/Fz.FR);
    normLongTireForce.RL = (Fx.RL/Fz.RL);
    normLongTireForce.RR = (Fx.RR/Fz.RR);

%     %Front left
%     if (SR.FL > mu_lo_slip_lim) && (SR.FL < mu_hi_slip_lim)
%         mu_FL = (1-mu_forget_factor)*mu_FL + mu_forget_factor*normLongTireForce.FL;
%     elseif (SR.FL > mu_no_slip_lim) && (SR.FL < mu_lo_slip_lim)
%         mu_FL = (1-mu_forget_factor)*mu_FL + mu_growth_factor;
%     elseif (SR.FL > mu_lo_slip_lim) && (SR.FL < mu_full_slip_lim)
%         mu_FL = (1-mu_forget_factor)*mu_FL - mu_shrink_factor;        
%     end
%     %Front right
%     if (SR.FR > mu_lo_slip_lim) && (SR.FR < mu_hi_slip_lim)
%         mu_FR = (1-mu_forget_factor)*mu_FR + mu_forget_factor*normLongTireForce.FR;
%     elseif (SR.FR > mu_no_slip_lim) && (SR.FR < mu_lo_slip_lim)
%         mu_FR = (1-mu_forget_factor)*mu_FR + mu_growth_factor;
%     elseif (SR.FR > mu_lo_slip_lim) && (SR.FR < mu_full_slip_lim)
%         mu_FR = (1-mu_forget_factor)*mu_FR - mu_shrink_factor;        
%     end
%     %Rear left
%     if ( SR.RL > mu_lo_slip_lim) && (SR.RL < mu_hi_slip_lim)
%         mu_RL = (1-mu_forget_factor)*mu_RL + mu_forget_factor*normLongTireForce.RL;
%     elseif (SR.RL > mu_no_slip_lim) && (SR.RL < mu_lo_slip_lim)
%         mu_RL = (1-mu_forget_factor)*mu_RL + mu_growth_factor;
%     elseif (SR.RL > mu_lo_slip_lim) && (SR.RL < mu_full_slip_lim)
%         mu_RL = (1-mu_forget_factor)*mu_RL - mu_shrink_factor;        
%     end
%     %Rear right
%     if (SR.RR > mu_lo_slip_lim) && (SR.RR < mu_hi_slip_lim)
%        mu_RR = (1-mu_forget_factor)*mu_RR + mu_forget_factor*normLongTireForce.RR;
%     elseif (SR.RR > mu_no_slip_lim) && (SR.RR < mu_lo_slip_lim)
%        mu_RR = (1-mu_forget_factor)*mu_RR + mu_growth_factor;
%     elseif (SR.RR > mu_lo_slip_lim) && (SR.RR < mu_full_slip_lim)
%        mu_RR = (1-mu_forget_factor)*mu_RR - mu_shrink_factor;        
%     end
%}
end

mu = settings.mu;
mu_estimate = 0.25*(mu_FL+mu_FR+mu_RL+mu_RR);

end

== matlab function TV_2017/CarMaker/Estimations/Fz_estimators/Fz_Estimation/1st_deriv/Diff_Function ==
  data: y_old output; y_old input; sig input; y output; delta_t input
function [y_old,y] = innerFunction(y_old, sig, delta_t)

y_old = circshift(y_old,1);
y_old(1) = sig;
        
M = length(y_old);
N = 3;
nu = 1;
j = 1;

k = 1:M;

x = phi(M,N,nu,j,k,delta_t) .* y_old;

y = sum(x);

end

function p = phi(M,N,nu,j,k,delta_t)

fac = (factorial(N + j + nu + 1) .*...
    factorial(N + 1)) ./...
    (M .* delta_t) .^ j;

[i,k2,k1,k] = ndgrid(0:nu + N,0:j,0:N-j,k);

eliminator = i > nu + k1 + k2;

evalIn = inPhi(M,N,nu,j,k,i,k1,k2);
evalIn(eliminator) = 0;

p = fac * sum(sum(sum(evalIn)));

p = p(:);

end

function p = inPhi(M,N,nu,j,k,i,k1,k2)

p = ((-1).^(N + i - k1 - k2) .*...
    ((k./M).^(N + i - k1 - k2 + 1) - ...
    ((k-1)./M).^(N + i - k1 - k2 + 1)))./...
    (factorial(k1) .* factorial(k2) .* factorial(i).*...
    factorial(N - j - k1) .*...
    factorial(j - k2) .*...
    factorial(N - k1 - k2) .*...
    factorial(nu - i + k1 + k2) .*...
    (N - k1 + 1) .*...
    (N + i -k1 - k2 + 1));

end

function n = factorial(n)

fac = [1;1;2;6;24;120;720;5040;40320;362880;3628800;39916800;479001600;6227020800.00000;87178291200.0000;1307674368000.00;20922789888000.0;355687428096000;6.40237370572800e+15;1.21645100408832e+17;2.43290200817664e+18;5.10909421717094e+19;1.12400072777761e+21;2.58520167388850e+22;6.20448401733239e+23;1.55112100433310e+25;4.03291461126606e+26;1.08888694504184e+28;3.04888344611714e+29;8.84176199373970e+30;2.65252859812191e+32;8.22283865417792e+33;2.63130836933694e+35;8.68331761881189e+36;2.95232799039604e+38;1.03331479663861e+40;3.71993326789901e+41;1.37637530912263e+43;5.23022617466601e+44;2.03978820811974e+46;8.15915283247898e+47;3.34525266131638e+49;1.40500611775288e+51;6.04152630633738e+52;2.65827157478845e+54;1.19622220865480e+56;5.50262215981209e+57;2.58623241511168e+59;1.24139155925361e+61;6.08281864034268e+62;3.04140932017134e+64];
n(n<0) = 0;
n = fac(n + 1);

end

== matlab function TV_2017/CarMaker/Estimations/Fz_estimators/Fz_Estimation/2nd_deriv/Diff_Function ==
  data: y_old output; y_old input; sig input; y output; delta_t input
function [y_old,y] = innerFunction(y_old, sig, delta_t)

y_old = circshift(y_old,1);
y_old(1) = sig;
        
M = length(y_old);
N = 3;
nu = 0;
j = 2;

k = 1:M;

x = phi(M,N,nu,j,k,delta_t) .* y_old;

y = sum(x);

end

function p = phi(M,N,nu,j,k,delta_t)

fac = (factorial(N + j + nu + 1) .*...
    factorial(N + 1)) ./...
    (M .* delta_t) .^ j;

[i,k2,k1,k] = ndgrid(0:nu + N,0:j,0:N-j,k);

eliminator = i > nu + k1 + k2;

evalIn = inPhi(M,N,nu,j,k,i,k1,k2);
evalIn(eliminator) = 0;

p = fac * sum(sum(sum(evalIn)));

p = p(:);

end

function p = inPhi(M,N,nu,j,k,i,k1,k2)

p = ((-1).^(N + i - k1 - k2) .*...
    ((k./M).^(N + i - k1 - k2 + 1) - ...
    ((k-1)./M).^(N + i - k1 - k2 + 1)))./...
    (factorial(k1) .* factorial(k2) .* factorial(i).*...
    factorial(N - j - k1) .*...
    factorial(j - k2) .*...
    factorial(N - k1 - k2) .*...
    factorial(nu - i + k1 + k2) .*...
    (N - k1 + 1) .*...
    (N + i -k1 - k2 + 1));

end

function n = factorial(n)

fac = [1;1;2;6;24;120;720;5040;40320;362880;3628800;39916800;479001600;6227020800.00000;87178291200.0000;1307674368000.00;20922789888000.0;355687428096000;6.40237370572800e+15;1.21645100408832e+17;2.43290200817664e+18;5.10909421717094e+19;1.12400072777761e+21;2.58520167388850e+22;6.20448401733239e+23;1.55112100433310e+25;4.03291461126606e+26;1.08888694504184e+28;3.04888344611714e+29;8.84176199373970e+30;2.65252859812191e+32;8.22283865417792e+33;2.63130836933694e+35;8.68331761881189e+36;2.95232799039604e+38;1.03331479663861e+40;3.71993326789901e+41;1.37637530912263e+43;5.23022617466601e+44;2.03978820811974e+46;8.15915283247898e+47;3.34525266131638e+49;1.40500611775288e+51;6.04152630633738e+52;2.65827157478845e+54;1.19622220865480e+56;5.50262215981209e+57;2.58623241511168e+59;1.24139155925361e+61;6.08281864034268e+62;3.04140932017134e+64];
n(n<0) = 0;
n = fac(n + 1);

end

== matlab function TV_2017/CarMaker/Control_System /Slip Rate Control /Traction Controllers/MATLAB Function ==
  data: Ti_FL input; Ti_FR input; Ti_lim output Bus: Ti_lim; Ti_RL input; Ti_RR input; TC_FL input; TC_FR input; TC_RL input; TC_RR input; states input Bus: States; T_req input
function Ti_lim =  TCOutputHandling(Ti_FL, Ti_FR, Ti_RL, Ti_RR, TC_FL,TC_FR,TC_RL,TC_RR,states, T_req)
%#codegen


Ti_lim.FL = Ti_FL + TC_FL;
Ti_lim.FR = Ti_FR + TC_FR;
Ti_lim.RL = Ti_RL + TC_RL;
Ti_lim.RR = Ti_RR + TC_RR;


% yawRate_p_lim = 0.3;
% ay_p_lim = 3;
% 
% straightline = uint32(0);
% 
% if ( (states.r > -yawRate_p_lim) && (states.r < yawRate_p_lim) &&...
%      (states.ay > -ay_p_lim) && (states.ay < ay_p_lim) )
%     straightline = 1;
% else
%     straightline = 0;
% end
% 
% 
% % FRONT SIDE
% n_cmp = single(-0.03);
% p_cmp = single(0.03);
% 
% % If driving ~ straightline then couple the outputs
% % Else, each TC works individually. 
% if      ( (straightline == 1) && (T_req > p_cmp) )
%     % Couple TC outputs to maintain stability on mu split surfaces 
%     % under acceleration and deceleration
%     Ti_lim.FL = max(0, (Ti_FL + min(TC_FL,TC_FR)));
%     Ti_lim.FR = max(0, (Ti_FR + min(TC_FL,TC_FR)));  
%     
%     Ti_lim.RL = max(0, (Ti_RL + min(TC_RL,TC_RR)));
%     Ti_lim.RR = max(0, (Ti_RR + min(TC_RL,TC_RR)));
%  
% elseif  ( (straightline == 1) && (T_req < n_cmp) )
%     % Couple TC outputs to maintain stability on mu split surfaces 
%     % under acceleration and deceleration
%     Ti_lim.FL = min(0, (Ti_FL + max(TC_FL,TC_FR) ) );   
%     Ti_lim.FR = min(0, (Ti_FR + max(TC_FL,TC_FR) ) );    
%     Ti_lim.RL = min(0, (Ti_RL + max(TC_RL,TC_RR) ) );
%     Ti_lim.RR = min(0, (Ti_RR + max(TC_RL,TC_RR) ) );   
% else
%     % Decouple TC outputs to avoid interferring too much with the stability
%     % of the vehicle while cornering. This is the DYC systems job. 
%     Ti_lim.FL = Ti_FL + TC_FL;
%     Ti_lim.FR = Ti_FR + TC_FR;
%     Ti_lim.RL = Ti_RL + TC_RL;
%     Ti_lim.RR = Ti_RR + TC_RR;
% end

end
